simulink model "photothermal"  (R2020b)
settings: Solver=VariableStepAuto  StartTime=0.0  StopTime=3e5  RelTol=1e-3  AbsTol=1e-3
PreLoadFcn:
  | pipe_area = 0.01; % m^2
  | furnace_temperature = 1500; % degC
  | boiler_liquid_level = 0.7; % 1
  | condenser_liquid_level = 0.2;
  | preheat_condenser_liquid_level = 0.2; % 1
undefined symbols (not defined in the file): sigbuilder_block
libraries: fl_lib x50, nesl_utility x18, RankineCycle_lib x5, pid_lib x2
(part 3 of 3)

== system photothermal/Subsystem/Check Valve ==
  Pressure & Internal Energy Sensor (2P) : fl_lib/Two-Phase Fluid/Sensors/Pressure & Internal Energy Sensor (2P)
      settings: SourceProductName=Foundation Library  InternalSimscapePortConfiguration="{\"Bottom\":[],\"Left\":[{\"id\":\"A\",\"label\":\"A\",\"type\":\"foundation.two_phase_fluid.two_phase_fluid\"}],\"Right\":[{\"id\":\"B\",\"label\":\"B\",\"type\":\"foundation.two_phase_fluid.two_phase_fluid\"},{\"id\":\"P\",\"label\":\"P\",\"type\":\"output\"},{\"id\":\"U\",\"label\":\"U\",\"type\":\"output\"}],\"Top\":[]}"
  Valve Gain : Subsystem
  Variable Local Restriction (2P) : fl_lib/Two-Phase Fluid/Elements/Variable Local Restriction (2P)  min_area=min_area m^2  max_area=max_area m^2  area=pipe_area m^2  Cd=Cd  B_lam=0.999
      settings: SourceProductName=Foundation Library  InternalSimscapePortConfiguration="{\"Bottom\":[],\"Left\":[{\"id\":\"A\",\"label\":\"A\",\"type\":\"foundation.two_phase_fluid.two_phase_fluid\"},{\"id\":\"area_in\",\"label\":\"AR\",\"type\":\"input\"}],\"Right\":[{\"id\":\"B\",\"label\":\"B\",\"type\":\"foundation.two_phase_fluid.two_phase_fluid\"}],\"Top\":[]}"
  A : PMIOPort  Side=Left
  B : PMIOPort  Port=2  Side=Right
  connections:
  Pressure & Internal Energy Sensor (2P)/LConn1 -- Variable Local Restriction (2P)/LConn1 -- A/RConn1
  Variable Local Restriction (2P)/RConn1 -- B/RConn1 -- Pressure & Internal Energy Sensor (2P)/RConn1
  Valve Gain/LConn1 -- Pressure & Internal Energy Sensor (2P)/RConn2
  Valve Gain/RConn1 -- Variable Local Restriction (2P)/LConn2

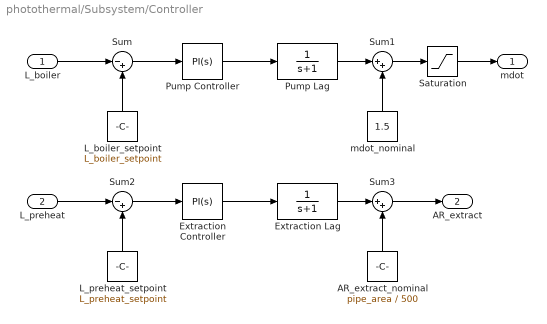
== system photothermal/Subsystem/Controller ==
  L_boiler : Inport
  L_preheat : Inport  Port=2
  AR_extract_nominal : Constant  Value=pipe_area / 500
  Extraction Controller : pid_lib/PID Controller  Controller=PI  Form=Ideal  TimeDomain=Continuous-time  UseExternalTs=off  SampleTime=-1  IntegratorMethod=Forward Euler  FilterMethod=Forward Euler  ControllerParametersSource=internal  P=-0.01  I=0.01  D=0  UseFilter=on  N=100  TunerSelectOption=Transfer Function Based (PID Tuner App)  InitialConditionSource=internal  InitialConditionForIntegrator=0  InitialConditionForFilter=0  DifferentiatorICPrevScaledInput=0  ExternalReset=none  TrackingMode=off  Kt=1  LimitOutput=on  SatLimitsSource=internal  UpperSaturationLimit=pipe_area * (1/10 - 1/500)  LowerSaturationLimit=- pipe_area / 500  LinearizeAsGain=on  AntiWindupMode=back-calculation  Kb=1  POutMin=[]  POutMax=[]  IOutMin=[]  IOutMax=[]  DOutMin=[]  DOutMax=[]  NOutMin=[]  NOutMax=[]  SumOutMin=[]  SumOutMax=[]  SaturationOutMin=[]  SaturationOutMax=[]  PParamMin=[]  PParamMax=[]  IParamMin=[]  IParamMax=[]  DParamMin=[]  DParamMax=[]  NParamMin=[]  NParamMax=[]  KbParamMin=[]  KbParamMax=[]  KtParamMin=[]  KtParamMax=[]  KbOutMin=[]  KbOutMax=[]  KtOutMin=[]  KtOutMax=[]  IntegratorOutMin=[]  IntegratorOutMax=[]  FilterOutMin=[]  FilterOutMax=[]  SumI1OutMin=[]  SumI1OutMax=[]  SumI2OutMin=[]  SumI2OutMax=[]  SumI3OutMin=[]  SumI3OutMax=[]  SumI4OutMin=[]  SumI4OutMax=[]  SumDOutMin=[]  SumDOutMax=[]  DifferentiatorOutMin=[]  DifferentiatorOutMax=[]  FilterDiffOutCoefMin=[]  FilterDiffOutCoefMax=[]  ReciprocalOutMin=[]  ReciprocalOutMax=[]  SumDenOutMin=[]  SumDenOutMax=[]  SumNumOutMin=[]  SumNumOutMax=[]  DivideOutMin=[]  DivideOutMax=[]  UdiffTsProdOutMin=[]  UdiffTsProdOutMax=[]  NTsProdOutMin=[]  NTsProdOutMax=[]  UintegralTsProdOutMin=[]  UintegralTsProdOutMax=[]  UngainTsProdOutMin=[]  UngainTsProdOutMax=[]  IntegratorContinuousStateAttributes=''  IntegratorStateMustResolveToSignalObject=off  IntegratorRTWStateStorageClass=Auto  FilterContinuousStateAttributes=''  FilterStateMustResolveToSignalObject=off  FilterRTWStateStorageClass=Auto  ParallelPVariant=Passthrough  IdealPVariant=InternalParameters  IVariant=InternalParameters  DVariant=Disabled  IntegratorVariant=Continuous  SatVariant=Enabled  AWVariant=BackCalculation  PCopyVariant=Disabled  TRVariant=Disabled  FdbkBlocksVariant=Forward  IdealPFdbkVariant=Disabled  SatFdbkVariant=Disabled  DerivativeFilterVariant=Disabled  NVariant=Disabled  NCopyVariant=Disabled_SignalSpec  FilterICVariant=Disabled  IntegratorICVariant=InternalICs  ExternalResetVariant=Disabled  TRSumVariant=Passthrough  SumFdbkVariant=Disabled  SumVariant=Sum_PI  TsampFilterVariant=InternalTs  TsampNgainVariant=Passthrough  TsampIntegralVariant=Passthrough  ExternalSaturationOutDataTypeStr=Inherit: Same as second input
  Extraction Lag : TransferFcn  Denominator=[1 1]
  L_boiler_setpoint : Constant  Value=L_boiler_setpoint
  L_preheat_setpoint : Constant  Value=L_preheat_setpoint
  Pump Controller : pid_lib/PID Controller  Controller=PI  Form=Ideal  TimeDomain=Continuous-time  UseExternalTs=off  SampleTime=-1  IntegratorMethod=Forward Euler  FilterMethod=Forward Euler  ControllerParametersSource=internal  P=100  I=1e-4  D=0  UseFilter=on  N=100  TunerSelectOption=Transfer Function Based (PID Tuner App)  InitialConditionSource=internal  InitialConditionForIntegrator=0  InitialConditionForFilter=0  DifferentiatorICPrevScaledInput=0  ExternalReset=none  TrackingMode=off  Kt=1  LimitOutput=on  SatLimitsSource=internal  UpperSaturationLimit=20  LowerSaturationLimit=-1.5  LinearizeAsGain=on  AntiWindupMode=back-calculation  Kb=1  POutMin=[]  POutMax=[]  IOutMin=[]  IOutMax=[]  DOutMin=[]  DOutMax=[]  NOutMin=[]  NOutMax=[]  SumOutMin=[]  SumOutMax=[]  SaturationOutMin=[]  SaturationOutMax=[]  PParamMin=[]  PParamMax=[]  IParamMin=[]  IParamMax=[]  DParamMin=[]  DParamMax=[]  NParamMin=[]  NParamMax=[]  KbParamMin=[]  KbParamMax=[]  KtParamMin=[]  KtParamMax=[]  KbOutMin=[]  KbOutMax=[]  KtOutMin=[]  KtOutMax=[]  IntegratorOutMin=[]  IntegratorOutMax=[]  FilterOutMin=[]  FilterOutMax=[]  SumI1OutMin=[]  SumI1OutMax=[]  SumI2OutMin=[]  SumI2OutMax=[]  SumI3OutMin=[]  SumI3OutMax=[]  SumI4OutMin=[]  SumI4OutMax=[]  SumDOutMin=[]  SumDOutMax=[]  DifferentiatorOutMin=[]  DifferentiatorOutMax=[]  FilterDiffOutCoefMin=[]  FilterDiffOutCoefMax=[]  ReciprocalOutMin=[]  ReciprocalOutMax=[]  SumDenOutMin=[]  SumDenOutMax=[]  SumNumOutMin=[]  SumNumOutMax=[]  DivideOutMin=[]  DivideOutMax=[]  UdiffTsProdOutMin=[]  UdiffTsProdOutMax=[]  NTsProdOutMin=[]  NTsProdOutMax=[]  UintegralTsProdOutMin=[]  UintegralTsProdOutMax=[]  UngainTsProdOutMin=[]  UngainTsProdOutMax=[]  IntegratorContinuousStateAttributes=''  IntegratorStateMustResolveToSignalObject=off  IntegratorRTWStateStorageClass=Auto  FilterContinuousStateAttributes=''  FilterStateMustResolveToSignalObject=off  FilterRTWStateStorageClass=Auto  ParallelPVariant=Passthrough  IdealPVariant=InternalParameters  IVariant=InternalParameters  DVariant=Disabled  IntegratorVariant=Continuous  SatVariant=Enabled  AWVariant=BackCalculation  PCopyVariant=Disabled  TRVariant=Disabled  FdbkBlocksVariant=Forward  IdealPFdbkVariant=Disabled  SatFdbkVariant=Disabled  DerivativeFilterVariant=Disabled  NVariant=Disabled  NCopyVariant=Disabled_SignalSpec  FilterICVariant=Disabled  IntegratorICVariant=InternalICs  ExternalResetVariant=Disabled  TRSumVariant=Passthrough  SumFdbkVariant=Disabled  SumVariant=Sum_PI  TsampFilterVariant=InternalTs  TsampNgainVariant=Passthrough  TsampIntegralVariant=Passthrough  ExternalSaturationOutDataTypeStr=Inherit: Same as second input
  Pump Lag : TransferFcn  Denominator=[1 1]
  Saturation : Saturate  UpperLimit=30  LowerLimit=0
  Sum : Sum  Inputs=|-+
  Sum1 : Sum  Inputs=|++
  Sum2 : Sum  Inputs=|-+
  Sum3 : Sum  Inputs=|++
  mdot_nominal : Constant  Value=1.5
  mdot : Outport  VectorParamsAs1DForOutWhenUnconnected=off
  AR_extract : Outport  Port=2  VectorParamsAs1DForOutWhenUnconnected=off
  wires:
  L_boiler/1 -> Sum/1
  L_boiler_setpoint/1 -> Sum/2
  Sum/1 -> Pump Controller/1
  mdot_nominal/1 -> Sum1/2
  Pump Controller/1 -> Pump Lag/1
  Sum1/1 -> Saturation/1
  Sum3/1 -> AR_extract/1
  L_preheat_setpoint/1 -> Sum2/2
  L_preheat/1 -> Sum2/1
  AR_extract_nominal/1 -> Sum3/2
  Sum2/1 -> Extraction Controller/1
  Pump Lag/1 -> Sum1/1
  Extraction Lag/1 -> Sum3/1
  Extraction Controller/1 -> Extraction Lag/1
  Saturation/1 -> mdot/1

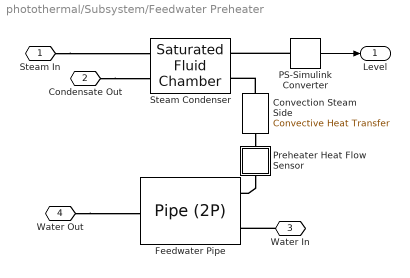
== system photothermal/Subsystem/Feedwater Preheater ==
  Convection Steam Side : fl_lib/Thermal/Thermal Elements/Convective Heat Transfer  area=pi * sqrt(4*pipe_area/pi) * pipe_length + fin_area m^2  heat_tr_coeff=steam_heat_coeff W/(m^2 * K)  T_specify=off  T_priority=None  T=0 K  T_nominal_specify=off  T_nominal_unit=K  T_nominal_value=1  Q_specify=off  Q_priority=None  Q=0 W  Q_nominal_specify=off  Q_nominal_unit=W  Q_nominal_value=1
      settings: SourceProductName=Foundation Library
  Feedwater Pipe : fl_lib/Two-Phase Fluid/Elements/Pipe (2P)  length=pipe_length m  area=pipe_area m^2  Dh=sqrt(4*pipe_area/pi) m  length_add=0.1 * pipe_length m  roughness=15e-6 m  Re_lam=2000  Re_tur=4000  shape_factor=64  Nu_lam=3.66  inertia=0  energy_spec=foundation.enum.energy_spec.temperature  p_init=p_water_init MPa  T_init=T_water_init degC  x_init=0.2  alpha_init=0.5  h_init=1500 kJ/kg  u_init=1500 kJ/kg  mdot_init=0 kg/s  time_constant=0.1 s
      settings: SourceProductName=Foundation Library  InternalSimscapePortConfiguration="{\"Bottom\":[],\"Left\":[{\"id\":\"A\",\"label\":\"A\",\"type\":\"foundation.two_phase_fluid.two_phase_fluid\"},{\"id\":\"H\",\"label\":\"H\",\"type\":\"foundation.thermal.thermal\"}],\"Right\":[{\"id\":\"B\",\"label\":\"B\",\"type\":\"foundation.two_phase_fluid.two_phase_fluid\"}],\"Top\":[]}"
  PS-Simulink Converter : nesl_utility/PS-Simulink Converter  PhysicalDomain=network_engine_domain  SubClassName=ps_output  LeftPortType=input  RightPortType=output  PseudoPeriodic=off  Frequencies=[]  Unit=1  AffineConversion=off
      settings: SourceProductName=Utilities
  Preheater Heat Flow Sensor : Subsystem
  Steam Condenser : RankineCycle_lib/Saturated Fluid Chamber  volume=condenser_volume m^3  area_A=pipe_area m^2  area_B=pipe_area m^2  L_min=0.01  L_max=0.99  p_I_specify=on  p_I_priority=High  p_I=p_steam_init MPa  p_I_nominal_specify=off  p_I_nominal_unit=MPa  p_I_nominal_value=1  L_specify=on  L_priority=High  L=L_init  L_nominal_specify=off  L_nominal_unit=1  L_nominal_value=1
      settings: SourceProductBaseCode=SS  InternalSimscapePortConfiguration="{\"Bottom\":[],\"Left\":[{\"id\":\"A\",\"label\":\"A\",\"type\":\"foundation.two_phase_fluid.two_phase_fluid\"},{\"id\":\"B\",\"label\":\"B\",\"type\":\"foundation.two_phase_fluid.two_phase_fluid\"}],\"Right\":[{\"id\":\"L_out\",\"label\":\"L\",\"type\":\"output\"},{\"id\":\"H\",\"label\":\"H\",\"type\":\"foundation.thermal.thermal\"}],\"Top\":[]}"
  Steam In : PMIOPort  Side=Left
  Condensate Out : PMIOPort  Port=2  Side=Right
  Water In : PMIOPort  Port=3  Side=Right
  Water Out : PMIOPort  Port=4  Side=Left
  Level : Outport  VectorParamsAs1DForOutWhenUnconnected=off
  wires:
  PS-Simulink Converter/1 -> Level/1
  connections:
  Water In/RConn1 -- Feedwater Pipe/LConn1
  Water Out/RConn1 -- Feedwater Pipe/RConn1
  Steam In/RConn1 -- Steam Condenser/LConn1
  Condensate Out/RConn1 -- Steam Condenser/LConn2
  Preheater Heat Flow Sensor/RConn1 -- Feedwater Pipe/LConn2
  PS-Simulink Converter/LConn1 -- Steam Condenser/RConn1
  Convection Steam Side/RConn1 -- Preheater Heat Flow Sensor/LConn1
  Convection Steam Side/LConn1 -- Steam Condenser/RConn2

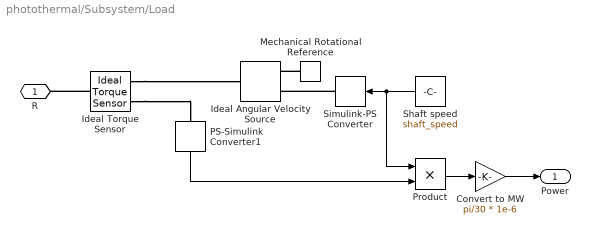
== system photothermal/Subsystem/Load ==
  Convert to MW : Gain  Gain=pi/30 * 1e-6
  Ideal Angular Velocity Source : fl_lib/Mechanical/Mechanical Sources/Ideal Angular Velocity Source
      settings: SourceProductName=Foundation Library
  Ideal Torque Sensor : fl_lib/Mechanical/Mechanical Sensors/Ideal Torque Sensor
      settings: SourceProductName=Foundation Library
  Mechanical Rotational Reference : fl_lib/Mechanical/Rotational Elements/Mechanical Rotational Reference
      settings: SourceProductName=Foundation Library
  PS-Simulink Converter1 : nesl_utility/PS-Simulink Converter  PhysicalDomain=network_engine_domain  SubClassName=ps_output  LeftPortType=input  RightPortType=output  PseudoPeriodic=off  Frequencies=[]  Unit=N*m  AffineConversion=off
      settings: SourceProductName=Utilities
  Product : Product
  Shaft speed : Constant  Value=shaft_speed
  Simulink-PS Converter : nesl_utility/Simulink-PS Converter  PhysicalDomain=network_engine_domain  SubClassName=ps_input  LeftPortType=input  RightPortType=output  PseudoPeriodic=off  Frequencies=[]  NoiseDistribution=none  NoiseParameters=[]  Unit=rpm  AffineConversion=off  FilteringAndDerivatives=provide  SimscapeFilterOrder=1  InputFilterTimeConstant=0.001  UdotUserProvided=0
      settings: SourceProductName=Utilities
  R : PMIOPort  Side=Left
  Power : Outport  VectorParamsAs1DForOutWhenUnconnected=off
  wires:
  Product/1 -> Convert to MW/1
  PS-Simulink Converter1/1 -> Product/2
  Shaft speed/1 -> Product/1, Simulink-PS Converter/1
  Convert to MW/1 -> Power/1
  connections:
  Mechanical Rotational Reference/LConn1 -- Ideal Angular Velocity Source/RConn2
  Ideal Torque Sensor/LConn1 -- R/RConn1
  Ideal Torque Sensor/RConn1 -- Ideal Angular Velocity Source/LConn1
  Simulink-PS Converter/RConn1 -- Ideal Angular Velocity Source/RConn1
  Ideal Torque Sensor/RConn2 -- PS-Simulink Converter1/LConn1

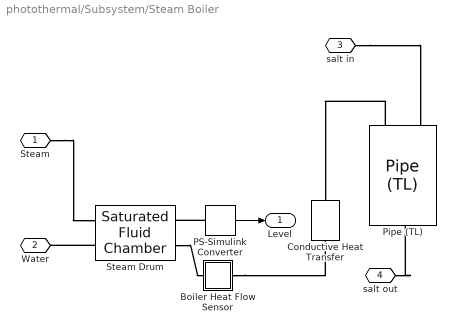
== system photothermal/Subsystem/Steam Boiler ==
  Boiler Heat Flow Sensor : Subsystem
  Conductive Heat Transfer : fl_lib/Thermal/Thermal Elements/Conductive Heat Transfer  area=1 m^2  thickness=0.1 m  th_cond=1000 W/(m*K)  T_specify=off  T_priority=None  T=0 K  T_nominal_specify=off  T_nominal_unit=K  T_nominal_value=1  Q_specify=off  Q_priority=None  Q=0 W  Q_nominal_specify=off  Q_nominal_unit=W  Q_nominal_value=1
  PS-Simulink Converter : nesl_utility/PS-Simulink Converter  PhysicalDomain=network_engine_domain  SubClassName=ps_output  LeftPortType=input  RightPortType=output  PseudoPeriodic=off  Frequencies=[]  Unit=1  AffineConversion=off
      settings: SourceProductName=Utilities
  Pipe (TL) : fl_lib/Thermal Liquid/Elements/Pipe (TL)  length=100 m  area=0.1 m^2  Dh=0.1128 m  length_add=1 m  roughness=15e-6 m  Re_lam=2000  Re_tur=4000  shape_factor=64  Nu_lam=3.66  dynamic_compressibility=simscape.enum.onoff.on  inertia=simscape.enum.onoff.off  p0=0.101325 MPa  T0=426 degC  mdot0=0 kg/s
      settings: SourceProductBaseCode=SS
  Steam Drum : RankineCycle_lib/Saturated Fluid Chamber  volume=boiler_volume m^3  area_A=pipe_area m^2  area_B=pipe_area m^2  L_min=0.01  L_max=0.99  p_I_specify=on  p_I_priority=High  p_I=p_init MPa  p_I_nominal_specify=off  p_I_nominal_unit=MPa  p_I_nominal_value=1  L_specify=on  L_priority=High  L=L_init  L_nominal_specify=off  L_nominal_unit=1  L_nominal_value=1
      settings: SourceProductBaseCode=SS  InternalSimscapePortConfiguration="{\"Bottom\":[],\"Left\":[{\"id\":\"A\",\"label\":\"A\",\"type\":\"foundation.two_phase_fluid.two_phase_fluid\"},{\"id\":\"B\",\"label\":\"B\",\"type\":\"foundation.two_phase_fluid.two_phase_fluid\"}],\"Right\":[{\"id\":\"L_out\",\"label\":\"L\",\"type\":\"output\"},{\"id\":\"H\",\"label\":\"H\",\"type\":\"foundation.thermal.thermal\"}],\"Top\":[]}"
  Steam : PMIOPort  Side=Left
  Water : PMIOPort  Port=2  Side=Left
  salt in : PMIOPort  Port=3  Side=Left
  salt out : PMIOPort  Port=4  Side=Left
  Level : Outport  VectorParamsAs1DForOutWhenUnconnected=off
  wires:
  PS-Simulink Converter/1 -> Level/1
  connections:
  Steam Drum/LConn2 -- Water/RConn1
  PS-Simulink Converter/LConn1 -- Steam Drum/RConn1
  Boiler Heat Flow Sensor/LConn1 -- Conductive Heat Transfer/RConn1
  Steam Drum/RConn2 -- Boiler Heat Flow Sensor/RConn1
  Steam/RConn1 -- Steam Drum/LConn1
  Pipe (TL)/LConn2 -- Conductive Heat Transfer/LConn1
  salt in/RConn1 -- Pipe (TL)/LConn1
  salt out/RConn1 -- Pipe (TL)/RConn1

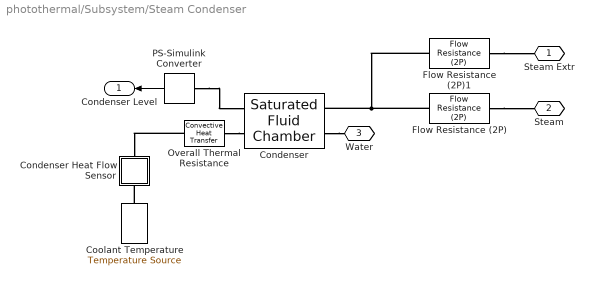
== system photothermal/Subsystem/Steam Condenser ==
  Condenser : RankineCycle_lib/Saturated Fluid Chamber  volume=condenser_volume m^3  area_A=pipe_area m^2  area_B=pipe_area m^2  L_min=0.01  L_max=0.99  p_I_specify=on  p_I_priority=High  p_I=p_init MPa  p_I_nominal_specify=off  p_I_nominal_unit=MPa  p_I_nominal_value=1  L_specify=on  L_priority=High  L=L_init  L_nominal_specify=off  L_nominal_unit=1  L_nominal_value=1
      settings: SourceProductBaseCode=SS  InternalSimscapePortConfiguration="{\"Bottom\":[],\"Left\":[{\"id\":\"A\",\"label\":\"A\",\"type\":\"foundation.two_phase_fluid.two_phase_fluid\"},{\"id\":\"B\",\"label\":\"B\",\"type\":\"foundation.two_phase_fluid.two_phase_fluid\"}],\"Right\":[{\"id\":\"L_out\",\"label\":\"L\",\"type\":\"output\"},{\"id\":\"H\",\"label\":\"H\",\"type\":\"foundation.thermal.thermal\"}],\"Top\":[]}"
  Condenser Heat Flow Sensor : Subsystem
  Coolant Temperature : fl_lib/Thermal/Thermal Sources/Temperature Source  temperature=T_coolant degC
      settings: SourceProductName=Foundation Library
  Flow Resistance (2P) : fl_lib/Two-Phase Fluid/Elements/Flow Resistance (2P)  delta_p_nominal=0.001 MPa  mdot_nominal=1.5 kg/s  v_nominal=0 m^3/kg  area=pipe_area * 2 m^2  laminar_fraction=1e-3
      settings: SourceProductName=Foundation Library  InternalSimscapePortConfiguration="{\"Bottom\":[],\"Left\":[{\"id\":\"A\",\"label\":\"A\",\"type\":\"foundation.two_phase_fluid.two_phase_fluid\"}],\"Right\":[{\"id\":\"B\",\"label\":\"B\",\"type\":\"foundation.two_phase_fluid.two_phase_fluid\"}],\"Top\":[]}"
  Flow Resistance (2P)1 : fl_lib/Two-Phase Fluid/Elements/Flow Resistance (2P)  delta_p_nominal=0.001 MPa  mdot_nominal=0.1 kg/s  v_nominal=0 m^3/kg  area=pipe_area m^2  laminar_fraction=1e-3
      settings: SourceProductName=Foundation Library  InternalSimscapePortConfiguration="{\"Bottom\":[],\"Left\":[{\"id\":\"A\",\"label\":\"A\",\"type\":\"foundation.two_phase_fluid.two_phase_fluid\"}],\"Right\":[{\"id\":\"B\",\"label\":\"B\",\"type\":\"foundation.two_phase_fluid.two_phase_fluid\"}],\"Top\":[]}"
  Overall Thermal Resistance : fl_lib/Thermal/Thermal Elements/Convective Heat Transfer  area=condenser_area m^2  heat_tr_coeff=condenser_heat_coeff W/(m^2 * K)  T_specify=off  T_priority=None  T=0 K  T_nominal_specify=off  T_nominal_unit=K  T_nominal_value=1  Q_specify=off  Q_priority=None  Q=0 W  Q_nominal_specify=off  Q_nominal_unit=W  Q_nominal_value=1
      settings: SourceProductName=Foundation Library
  PS-Simulink Converter : nesl_utility/PS-Simulink Converter  PhysicalDomain=network_engine_domain  SubClassName=ps_output  LeftPortType=input  RightPortType=output  PseudoPeriodic=off  Frequencies=[]  Unit=1  AffineConversion=off
      settings: SourceProductName=Utilities
  Steam Extr : PMIOPort  Side=Right
  Steam : PMIOPort  Port=2  Side=Right
  Water : PMIOPort  Port=3  Side=Right
  Condenser Level : Outport  VectorParamsAs1DForOutWhenUnconnected=off
  wires:
  PS-Simulink Converter/1 -> Condenser Level/1
  connections:
  Overall Thermal Resistance/RConn1 -- Condenser/RConn2
  Condenser/LConn2 -- Water/RConn1
  Coolant Temperature/LConn1 -- Condenser Heat Flow Sensor/RConn1
  Overall Thermal Resistance/LConn1 -- Condenser Heat Flow Sensor/LConn1
  Flow Resistance (2P)/RConn1 -- Flow Resistance (2P)1/RConn1 -- Condenser/LConn1
  Flow Resistance (2P)1/LConn1 -- Steam Extr/RConn1
  Flow Resistance (2P)/LConn1 -- Steam/RConn1
  PS-Simulink Converter/LConn1 -- Condenser/RConn1

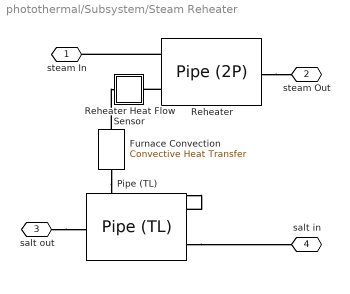
== system photothermal/Subsystem/Steam Reheater ==
  Furnace Convection : fl_lib/Thermal/Thermal Elements/Convective Heat Transfer  area=pi * sqrt(4*pipe_area/pi) * pipe_length + fin_area m^2  heat_tr_coeff=heater_heat_coeff W/(m^2 * K)  T_specify=off  T_priority=None  T=0 K  T_nominal_specify=off  T_nominal_unit=K  T_nominal_value=1  Q_specify=off  Q_priority=None  Q=0 W  Q_nominal_specify=off  Q_nominal_unit=W  Q_nominal_value=1
      settings: SourceProductName=Foundation Library
  Pipe (TL) : fl_lib/Thermal Liquid/Elements/Pipe (TL)  length=100 m  area=0.1 m^2  Dh=0.1128 m  length_add=1 m  roughness=15e-6 m  Re_lam=2000  Re_tur=4000  shape_factor=64  Nu_lam=3.66  dynamic_compressibility=simscape.enum.onoff.on  inertia=simscape.enum.onoff.off  p0=0.101325 MPa  T0=293.15 degC  mdot0=0 kg/s
      settings: SourceProductBaseCode=SS
  Reheater : fl_lib/Two-Phase Fluid/Elements/Pipe (2P)  length=pipe_length m  area=pipe_area m^2  Dh=sqrt(4*pipe_area/pi) m  length_add=0.1 * pipe_length m  roughness=15e-6 m  Re_lam=2000  Re_tur=4000  shape_factor=64  Nu_lam=3.66  inertia=0  energy_spec=foundation.enum.energy_spec.temperature  p_init=p_init MPa  T_init=T_init degC  x_init=0.2  alpha_init=0.5  h_init=1500 kJ/kg  u_init=1500 kJ/kg  mdot_init=0 kg/s  time_constant=0.1 s
      settings: SourceProductName=Foundation Library  InternalSimscapePortConfiguration="{\"Bottom\":[],\"Left\":[{\"id\":\"A\",\"label\":\"A\",\"type\":\"foundation.two_phase_fluid.two_phase_fluid\"},{\"id\":\"H\",\"label\":\"H\",\"type\":\"foundation.thermal.thermal\"}],\"Right\":[{\"id\":\"B\",\"label\":\"B\",\"type\":\"foundation.two_phase_fluid.two_phase_fluid\"}],\"Top\":[]}"
  Reheater Heat Flow Sensor : Subsystem
  steam In : PMIOPort  Side=Left
  steam Out : PMIOPort  Port=2  Side=Right
  salt out : PMIOPort  Port=3  Side=Left
  salt in : PMIOPort  Port=4  Side=Right
  connections:
  Reheater/LConn1 -- steam In/RConn1
  Reheater/RConn1 -- steam Out/RConn1
  Furnace Convection/LConn1 -- Pipe (TL)/LConn2
  Furnace Convection/RConn1 -- Reheater Heat Flow Sensor/LConn1
  Reheater/LConn2 -- Reheater Heat Flow Sensor/RConn1
  salt out/RConn1 -- Pipe (TL)/RConn1
  Pipe (TL)/LConn1 -- salt in/RConn1

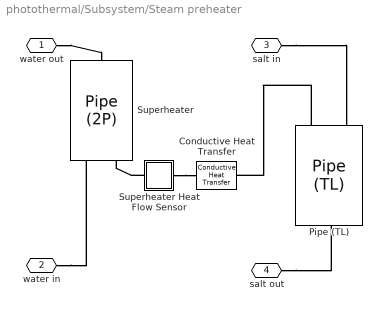
== system photothermal/Subsystem/Steam preheater ==
  Conductive Heat Transfer : fl_lib/Thermal/Thermal Elements/Conductive Heat Transfer  area=1e-4 m^2  thickness=0.1 m  th_cond=40000 W/(m*K)  T_specify=off  T_priority=None  T=0 K  T_nominal_specify=off  T_nominal_unit=K  T_nominal_value=1  Q_specify=off  Q_priority=None  Q=0 W  Q_nominal_specify=off  Q_nominal_unit=W  Q_nominal_value=1
  Pipe (TL) : fl_lib/Thermal Liquid/Elements/Pipe (TL)  length=5 m  area=0.1 m^2  Dh=0.1128 m  length_add=1 m  roughness=15e-6 m  Re_lam=2000  Re_tur=4000  shape_factor=64  Nu_lam=3.66  dynamic_compressibility=simscape.enum.onoff.on  inertia=simscape.enum.onoff.off  p0=0.101325 MPa  T0=293 degC  mdot0=0 kg/s
      settings: SourceProductBaseCode=SS
  Superheater : fl_lib/Two-Phase Fluid/Elements/Pipe (2P)  length=pipe_length m  area=pipe_area m^2  Dh=sqrt(4*pipe_area/pi) m  length_add=0.1 * pipe_length m  roughness=15e-6 m  Re_lam=2000  Re_tur=4000  shape_factor=64  Nu_lam=3.66  inertia=0  energy_spec=foundation.enum.energy_spec.temperature  p_init=p_init MPa  T_init=T_init degC  x_init=0.2  alpha_init=0.5  h_init=1500 kJ/kg  u_init=1500 kJ/kg  mdot_init=0 kg/s  time_constant=0.1 s
      settings: SourceProductName=Foundation Library  InternalSimscapePortConfiguration="{\"Bottom\":[],\"Left\":[{\"id\":\"A\",\"label\":\"A\",\"type\":\"foundation.two_phase_fluid.two_phase_fluid\"},{\"id\":\"H\",\"label\":\"H\",\"type\":\"foundation.thermal.thermal\"}],\"Right\":[{\"id\":\"B\",\"label\":\"B\",\"type\":\"foundation.two_phase_fluid.two_phase_fluid\"}],\"Top\":[]}"
  Superheater Heat Flow Sensor : Subsystem
  water out : PMIOPort  Side=Left
  "water in " : PMIOPort  Port=2  Side=Left
  salt in : PMIOPort  Port=3  Side=Left
  salt out : PMIOPort  Port=4  Side=Left
  connections:
  salt out/RConn1 -- Pipe (TL)/RConn1
  salt in/RConn1 -- Pipe (TL)/LConn1
  Pipe (TL)/LConn2 -- Conductive Heat Transfer/LConn1
  water out/RConn1 -- Superheater/RConn1
  Superheater Heat Flow Sensor/RConn1 -- Superheater/LConn2
  Superheater Heat Flow Sensor/LConn1 -- Conductive Heat Transfer/RConn1
  "water in "/RConn1 -- Superheater/LConn1

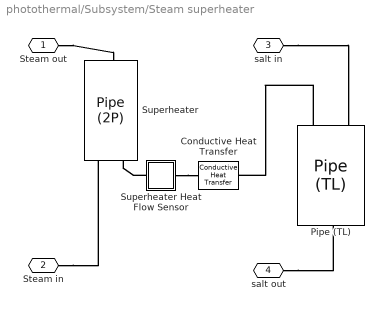
== system photothermal/Subsystem/Steam superheater ==
  Conductive Heat Transfer : fl_lib/Thermal/Thermal Elements/Conductive Heat Transfer  area=1e-4 m^2  thickness=0.1 m  th_cond=40000 W/(m*K)  T_specify=off  T_priority=None  T=0 K  T_nominal_specify=off  T_nominal_unit=K  T_nominal_value=1  Q_specify=off  Q_priority=None  Q=0 W  Q_nominal_specify=off  Q_nominal_unit=W  Q_nominal_value=1
  Pipe (TL) : fl_lib/Thermal Liquid/Elements/Pipe (TL)  length=100 m  area=0.1 m^2  Dh=0.1128 m  length_add=1 m  roughness=15e-6 m  Re_lam=2000  Re_tur=4000  shape_factor=64  Nu_lam=3.66  dynamic_compressibility=simscape.enum.onoff.on  inertia=simscape.enum.onoff.off  p0=0.101325 MPa  T0=540 degC  mdot0=0 kg/s
      settings: SourceProductBaseCode=SS
  Superheater : fl_lib/Two-Phase Fluid/Elements/Pipe (2P)  length=pipe_length m  area=pipe_area m^2  Dh=sqrt(4*pipe_area/pi) m  length_add=0.1 * pipe_length m  roughness=15e-6 m  Re_lam=2000  Re_tur=4000  shape_factor=64  Nu_lam=3.66  inertia=0  energy_spec=foundation.enum.energy_spec.temperature  p_init=p_init MPa  T_init=T_init degC  x_init=0.2  alpha_init=0.5  h_init=1500 kJ/kg  u_init=1500 kJ/kg  mdot_init=0 kg/s  time_constant=0.1 s
      settings: SourceProductName=Foundation Library  InternalSimscapePortConfiguration="{\"Bottom\":[],\"Left\":[{\"id\":\"A\",\"label\":\"A\",\"type\":\"foundation.two_phase_fluid.two_phase_fluid\"},{\"id\":\"H\",\"label\":\"H\",\"type\":\"foundation.thermal.thermal\"}],\"Right\":[{\"id\":\"B\",\"label\":\"B\",\"type\":\"foundation.two_phase_fluid.two_phase_fluid\"}],\"Top\":[]}"
  Superheater Heat Flow Sensor : Subsystem
  Steam out : PMIOPort  Side=Right
  "Steam in " : PMIOPort  Port=2  Side=Left
  salt in : PMIOPort  Port=3  Side=Left
  salt out : PMIOPort  Port=4  Side=Left
  connections:
  "Steam in "/RConn1 -- Superheater/LConn1
  Superheater Heat Flow Sensor/LConn1 -- Conductive Heat Transfer/RConn1
  Superheater Heat Flow Sensor/RConn1 -- Superheater/LConn2
  Steam out/RConn1 -- Superheater/RConn1
  Pipe (TL)/LConn2 -- Conductive Heat Transfer/LConn1
  salt in/RConn1 -- Pipe (TL)/LConn1
  salt out/RConn1 -- Pipe (TL)/RConn1

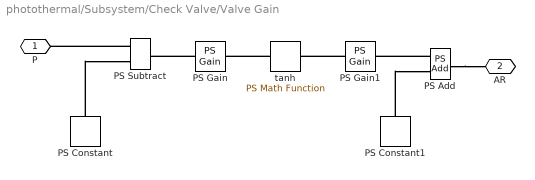
== system photothermal/Subsystem/Check Valve/Valve Gain ==
  PS Add : fl_lib/Physical Signals/Functions/PS Add
      settings: SourceProductName=Foundation Library
  PS Constant : fl_lib/Physical Signals/Sources/PS Constant  constant=(max_dp + min_dp) / 2 MPa
      settings: SourceProductName=Foundation Library
  PS Constant1 : fl_lib/Physical Signals/Sources/PS Constant  constant=(max_area + min_area) / 2 m^2
      settings: SourceProductName=Foundation Library
  PS Gain : fl_lib/Physical Signals/Functions/PS Gain  gain=6 / (max_dp - min_dp) 1/MPa
      settings: SourceProductName=Foundation Library
  PS Gain1 : fl_lib/Physical Signals/Functions/PS Gain  gain=(max_area - min_area) / 2 m^2
      settings: SourceProductName=Foundation Library
  PS Subtract : fl_lib/Physical Signals/Functions/PS Subtract
      settings: SourceProductName=Foundation Library
  tanh : fl_lib/Physical Signals/Functions/PS Math Function  fcn_choice=10
      settings: SourceProductName=Foundation Library
  P : PMIOPort  Side=Left
  AR : PMIOPort  Port=2  Side=Right
  connections:
  PS Add/LConn1 -- PS Gain1/RConn1
  PS Gain/LConn1 -- PS Subtract/RConn1
  PS Constant/RConn1 -- PS Subtract/LConn2
  PS Constant1/RConn1 -- PS Add/LConn2
  PS Subtract/LConn1 -- P/RConn1
  PS Add/RConn1 -- AR/RConn1
  tanh/LConn1 -- PS Gain/RConn1
  PS Gain1/LConn1 -- tanh/RConn1

== system photothermal/Subsystem/Feedwater Preheater/Preheater Heat Flow Sensor ==
  Heat Flow Rate Sensor : fl_lib/Thermal/Thermal Sensors/Heat Flow Rate Sensor
      settings: SourceProductName=Foundation Library
  A : PMIOPort  Side=Left
  B : PMIOPort  Port=2  Side=Right
  connections:
  Heat Flow Rate Sensor/RConn2 -- B/RConn1
  Heat Flow Rate Sensor/LConn1 -- A/RConn1

== system photothermal/Subsystem/Steam Boiler/Boiler Heat Flow Sensor ==
  Heat Flow Rate Sensor : fl_lib/Thermal/Thermal Sensors/Heat Flow Rate Sensor
      settings: SourceProductName=Foundation Library
  PS-Simulink Converter : nesl_utility/PS-Simulink Converter  PhysicalDomain=network_engine_domain  SubClassName=ps_output  LeftPortType=input  RightPortType=output  PseudoPeriodic=off  Frequencies=[]  Unit=MW  AffineConversion=off
      settings: SourceProductName=Utilities
  Scope : Scope  Commented=on
  A : PMIOPort  Side=Left
  B : PMIOPort  Port=2  Side=Right
  tag scope: Boiler=global
  wires:
  PS-Simulink Converter/1 -> [Boiler]
  connections:
  Heat Flow Rate Sensor/RConn2 -- B/RConn1
  Heat Flow Rate Sensor/LConn1 -- A/RConn1
  Heat Flow Rate Sensor/RConn1 -- PS-Simulink Converter/LConn1

== system photothermal/Subsystem/Steam Condenser/Condenser Heat Flow Sensor ==
  Heat Flow Rate Sensor : fl_lib/Thermal/Thermal Sensors/Heat Flow Rate Sensor
      settings: SourceProductName=Foundation Library
  A : PMIOPort  Side=Left
  B : PMIOPort  Port=2  Side=Right
  connections:
  Heat Flow Rate Sensor/RConn2 -- B/RConn1
  Heat Flow Rate Sensor/LConn1 -- A/RConn1

== system photothermal/Subsystem/Steam Reheater/Reheater Heat Flow Sensor ==
  Heat Flow Rate Sensor : fl_lib/Thermal/Thermal Sensors/Heat Flow Rate Sensor
      settings: SourceProductName=Foundation Library
  PS-Simulink Converter : nesl_utility/PS-Simulink Converter  PhysicalDomain=network_engine_domain  SubClassName=ps_output  LeftPortType=input  RightPortType=output  PseudoPeriodic=off  Frequencies=[]  Unit=MW  AffineConversion=off
      settings: SourceProductName=Utilities
  A : PMIOPort  Side=Left
  B : PMIOPort  Port=2  Side=Right
  tag scope: Reheater=global
  wires:
  PS-Simulink Converter/1 -> [Reheater]
  connections:
  Heat Flow Rate Sensor/RConn1 -- PS-Simulink Converter/LConn1
  Heat Flow Rate Sensor/LConn1 -- A/RConn1
  Heat Flow Rate Sensor/RConn2 -- B/RConn1

== system photothermal/Subsystem/Steam preheater/Superheater Heat Flow Sensor ==
  Heat Flow Rate Sensor : fl_lib/Thermal/Thermal Sensors/Heat Flow Rate Sensor
      settings: SourceProductName=Foundation Library
  PS-Simulink Converter : nesl_utility/PS-Simulink Converter  PhysicalDomain=network_engine_domain  SubClassName=ps_output  LeftPortType=input  RightPortType=output  PseudoPeriodic=off  Frequencies=[]  Unit=MW  AffineConversion=off
      settings: SourceProductName=Utilities
  A : PMIOPort  Side=Left
  B : PMIOPort  Port=2  Side=Right
  tag scope: Preheater=global
  wires:
  PS-Simulink Converter/1 -> [Preheater]
  connections:
  Heat Flow Rate Sensor/RConn2 -- B/RConn1
  Heat Flow Rate Sensor/LConn1 -- A/RConn1
  Heat Flow Rate Sensor/RConn1 -- PS-Simulink Converter/LConn1

== system photothermal/Subsystem/Steam superheater/Superheater Heat Flow Sensor ==
  Heat Flow Rate Sensor : fl_lib/Thermal/Thermal Sensors/Heat Flow Rate Sensor
      settings: SourceProductName=Foundation Library
  PS-Simulink Converter : nesl_utility/PS-Simulink Converter  PhysicalDomain=network_engine_domain  SubClassName=ps_output  LeftPortType=input  RightPortType=output  PseudoPeriodic=off  Frequencies=[]  Unit=MW  AffineConversion=off
      settings: SourceProductName=Utilities
  A : PMIOPort  Side=Left
  B : PMIOPort  Port=2  Side=Right
  tag scope: Superheat=global
  wires:
  PS-Simulink Converter/1 -> [Superheat]
  connections:
  Heat Flow Rate Sensor/RConn1 -- PS-Simulink Converter/LConn1
  Heat Flow Rate Sensor/LConn1 -- A/RConn1
  Heat Flow Rate Sensor/RConn2 -- B/RConn1
